simulink model "Heat_Exchanger"  (R2022b)
settings: Solver=VariableStepAuto  StartTime=0.0  StopTime=10.0  RelTol=1e-3
settings Model: Creator=Crapon  LastModifiedBy=Crapon

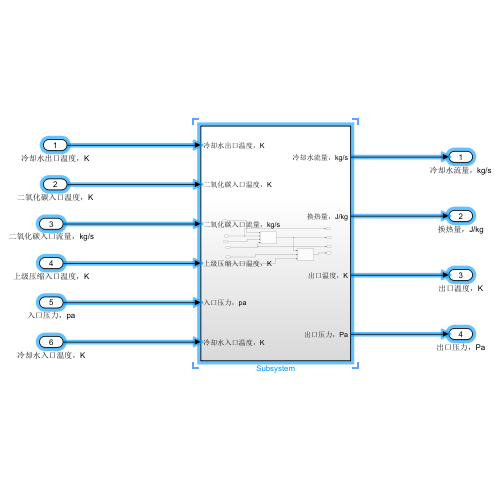
[thumbnail: Simulink's stored preview of the top-level diagram]
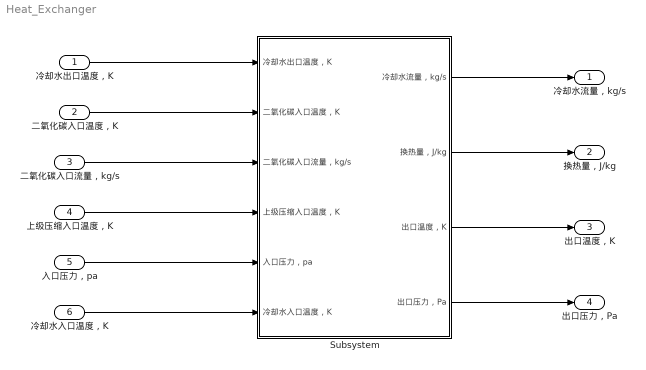
== system Heat_Exchanger ==
  冷却水出口温度，K : Inport
  二氧化碳入口温度，K : Inport  Port=2
  二氧化碳入口流量，kg/s : Inport  Port=3
  上级压缩入口温度，K : Inport  Port=4
  入口压力，pa : Inport  Port=5
  冷却水入口温度，K : Inport  Port=6
  Subsystem : Subsystem
  冷却水流量，kg/s : Outport
  换热量，J/kg : Outport  Port=2
  出口温度，K : Outport  Port=3
  出口压力，Pa : Outport  Port=4
  wires:
  冷却水出口温度，K/1 -> Subsystem/1(冷却水出口温度，K)
  二氧化碳入口温度，K/1 -> Subsystem/2(二氧化碳入口温度，K)
  二氧化碳入口流量，kg/s/1 -> Subsystem/3(二氧化碳入口流量，kg/s)
  上级压缩入口温度，K/1 -> Subsystem/4(上级压缩入口温度，K)
  入口压力，pa/1 -> Subsystem/5(入口压力，pa)
  冷却水入口温度，K/1 -> Subsystem/6(冷却水入口温度，K)
  Subsystem/1(冷却水流量，kg/s) -> 冷却水流量，kg/s/1
  Subsystem/2(换热量，J/kg) -> 换热量，J/kg/1
  Subsystem/3(出口温度，K) -> 出口温度，K/1
  Subsystem/4(出口压力，Pa) -> 出口压力，Pa/1

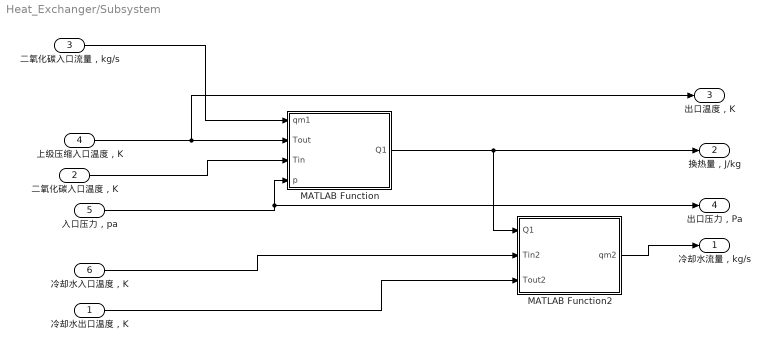
== system Heat_Exchanger/Subsystem ==
  冷却水出口温度，K : Inport
  二氧化碳入口温度，K : Inport  Port=2
  二氧化碳入口流量，kg/s : Inport  Port=3
  上级压缩入口温度，K : Inport  Port=4
  入口压力，pa : Inport  Port=5
  冷却水入口温度，K : Inport  Port=6
  MATLAB Function : MATLAB Function  TreatAsAtomicUnit=on
  MATLAB Function2 : MATLAB Function  TreatAsAtomicUnit=on
  冷却水流量，kg/s : Outport
  换热量，J/kg : Outport  Port=2
  出口温度，K : Outport  Port=3
  出口压力，Pa : Outport  Port=4
  wires:
  MATLAB Function/1(Q1) -> 换热量，J/kg/1, MATLAB Function2/1(Q1)
  冷却水出口温度，K/1 -> MATLAB Function2/3(Tout2)
  冷却水入口温度，K/1 -> MATLAB Function2/2(Tin2)
  MATLAB Function2/1(qm2) -> 冷却水流量，kg/s/1
  二氧化碳入口温度，K/1 -> MATLAB Function/3(Tin)
  上级压缩入口温度，K/1 -> 出口温度，K/1, MATLAB Function/2(Tout)
  二氧化碳入口流量，kg/s/1 -> MATLAB Function/1(qm1)
  入口压力，pa/1 -> MATLAB Function/4(p), 出口压力，Pa/1

== matlab function Heat_Exchanger/Subsystem/MATLAB Function ==
  data: qm1 input; Tout input; Tin input; Q1 output; p input
function Q1 = fc(qm1,Tout,Tin,p)
t=(Tin+Tout)/2;
cp=refpropm('C','T',t,'P',1000*p,'CO2');
Q1= qm1*cp*(Tout-Tin);

== matlab function Heat_Exchanger/Subsystem/MATLAB Function2 ==
  data: Q1 input; Tin2 input; Tout2 input; qm2 output
function qm2 = fcn(Q1,Tin2,Tout2)
t=(Tin2+Tout2)/2;
cp=refpropm('C','T',t,'Q',0,'water');
qm2= Q1/(cp*(Tout2-Tin2));
